simulink model "MSM_strain_wave_actuator"  (R2024b)
settings: Solver=ode23t  StartTime=0.0  StopTime=SIMULATION_TIME  FixedStep=MAX_TIME_STEP  MaxStep=MAX_TIME_STEP  RelTol=1e-3  AbsTol=1e-3  EnableMultiTasking=on
PreLoadFcn:
  | linear_mechanism = Simulink.Variant('motion_type == "linear"');
  | rotary_mechanism = Simulink.Variant('motion_type == "rotary"');
values from neighbouring files (symbols this model uses):
  action = round(out.position_data.Data(:,5))    [msm_tooth_training_run.m]
  contact_ratio = tooth_plates_cnt / (2 * (t_a / t_b + 1))    (= 2)    [MSM_mechanism_simulation_properties.m]
  contraction_initial = -msm_length * e_initial    (= -0.001)    [MSM_mechanism_simulation_properties.m]
  controller_type_vec = zeros(tooth_plates_cnt, 1)    [MSM_mechanism_simulation_properties.m]
  controller_velocity_setpoint = velocity_iter    [controller_mass_comparison_runs.m]
  disk_diameter = disk_teeth_count * tooth_pitch / pi    [MSM_mechanism_simulation_properties.m]    (also in msm_sim_runs_for_pid.m = evalin('base','disk_diameter'); save_sim_result.m = evalin('base','disk_diameter'))
  disk_height = 2.5e-4    (= 0.00025)    [MSM_mechanism_simulation_properties.m]    (also in get_tooth_properties.m)
  feedback_threshold = 1.025    [MSM_mechanism_simulation_properties.m]    (also in get_tooth_properties.m; msm_sim_runs_for_pid.m = evalin('base','feedback_threshold'))
  force_control_coeff = 1.0    (= 1)    [MSM_mechanism_simulation_properties.m]
  HALT_VELOCITY = 0.2    [MSM_mechanism_simulation_properties.m]    (also in get_tooth_properties.m)
  in_pair_angle_tooth_plates_pitch = 2*pi * (-2*tooth_pitch + in_pair_tooth_plates_pitch) / (pi*disk_diameter)    (= 0.412285714286)    [MSM_mechanism_simulation_properties.m]    (also in get_tooth_properties.m = 2*pi * (-2*tooth_pitch + in_pair_tooth_plates_pitch) / (pi*t)
  MAX_OVERLOAD_VELOCITY = 100    [MSM_mechanism_simulation_properties.m]    (also in get_tooth_properties.m)
  MAX_POSITION = rack_initial_position + max_teeth_passed * tooth_plates_cnt * angle_single_tooth_step    [MSM_mechanism_simulation_properties.m]    (also in get_tooth_properties.m)
  MAX_TIME_STEP = 5e-6    (= 5e-06)    [MSM_mechanism_simulation_properties.m]
  min_tooth_motion_range = -msm_length * allowed_elongation    (= -0.001)    [MSM_mechanism_simulation_properties.m]
  motion_type_number = NaN    [MSM_mechanism_simulation_properties.m]
  next_vec_fraction = -0.05    [MSM_mechanism_simulation_properties.m]    (also in msm_sim_runs_for_pid.m = evalin('base','next_vec_fraction'))
  obs_matrix = zeros(tooth_plates_cnt, obs_matrix_size)    [MSM_mechanism_simulation_properties.m]
  one_side_absolute_offset = one_side_elongation_capacity * msm_length    (= 0.0001)    [MSM_mechanism_simulation_properties.m]
  rack_coulumb_friction = 0.05    [MSM_mechanism_simulation_properties.m]
  rack_initial_position = rack_initial_position + 4*angle_single_tooth_step    (= 0.0554357142857)    [MSM_mechanism_simulation_properties.m]    (also in get_tooth_properties.m = rack_initial_position + 4*angle_single_tooth_step)
  rack_mass = 4e-3    (= 0.004)    [MSM_mechanism_simulation_properties.m]
  rotational_rack_coulumb_friction = rack_coulumb_friction * disk_diameter    (= 0.00175)    [MSM_mechanism_simulation_properties.m]
  SIMULATION_TIME = 0.06    [MSM_mechanism_simulation_properties.m]    (also in msm_actuation_time_sensetivity.m = 0.04; msm_sim_runs_for_pid.m = evalin('base','SIMULATION_TIME'); msm_simulation_run.m = 0.08; msm_tooth_training_run.m = 0.04)
  swing_block_tooth_plates_pitch = 2 * tooth_pitch * 22 + tooth_pitch / tooth_plates_cnt    (= 0.0172575)    [MSM_mechanism_simulation_properties.m]    (also in get_tooth_properties.m = 2 * tooth_pitch * 22 + tooth_pitch / tooth_plates_cnt)
  tooth_disk_mass = 5e-3    (= 0.005)    [MSM_mechanism_simulation_properties.m]
  tooth_pitch = tooth_pitch * tooth_size_modifier    (= 0.00039)    [MSM_mechanism_simulation_properties.m]    (also in get_tooth_properties.m = 0.00024661; msm_sim_runs_for_pid.m = evalin('base','tooth_pitch'); save_sim_result.m = evalin('base','tooth_pitch'))
  tooth_plates_cnt = 4    [MSM_mechanism_simulation_properties.m]    (also in MSM_simulation_data_processing.m = sim_data.tooth_plates_cnt; msm_actuation_time_sensetivity.m = plates_cnt_iter; msm_sim_runs_for_pid.m = evalin('base','tooth_plates_cnt'); msm_simulation_run.m = plates_cnt_iter)
  tooth_plates_pitch = tooth_pitch * 12 + tooth_pitch / tooth_plates_cnt    (= 0.0047775)    [MSM_mechanism_simulation_properties.m]    (also in get_tooth_properties.m = tooth_pitch * 12 + tooth_pitch / tooth_plates_cnt)
  useful_load = -2    [MSM_mechanism_simulation_properties.m]    (also in controller_mass_comparison_runs.m)
  useful_mass = 0.0001    [MSM_mechanism_simulation_properties.m]    (also in controller_mass_comparison_runs.m = 0.025)
  VALIDATION_START_TIME = 0.25*SIMULATION_TIME    (= 0.015)    [MSM_mechanism_simulation_properties.m]
  Z = griddata(x,y,z,X,Y)    [MSM_simulation_data_processing.m]
undefined symbols (not defined in the file or in its folder): controller_amplitude_setpoint, controller_desired_profile_type, controller_frequency_setpoint, controller_loop_type, enable_neighbours_obs, enable_vel_setpoint, external_control_value, has_external_controller, initial_spike_force, random_delay_probablity, random_switch_probability, sim_state_code, simulation_pause_time, X, Y
libraries: sm_lib x141, MSM_element x72, Flat_tooth_plate x36, Rotary_tooth_plate x36, Swing_mechanism x18, nesl_utility x16, simulink x10, fl_lib x9, rllib x7, spsMeanLib x2, slctrl_autotuning x2, slpidlib x1
(part 2 of 7)

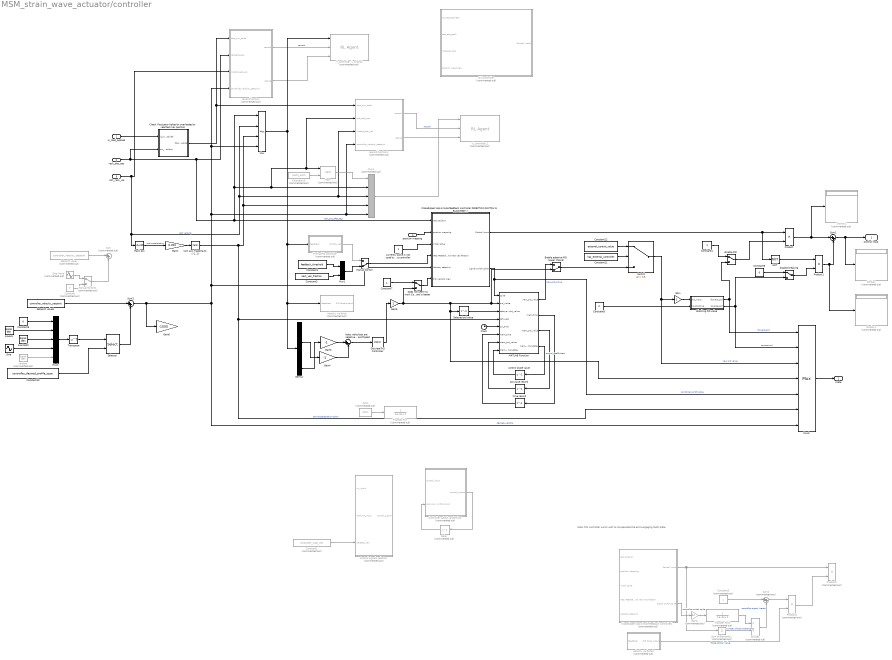
== system MSM_strain_wave_actuator/controller ==
  note: Note: this controller works well to compensate the extra engaging tooth plate
  is_load_applied : Inport
  rack_abs_pos : Inport  Port=2
  inst_rack_vel : Inport  Port=3
  position mapping : Inport  Port=4
  Blocking PID value : MATLAB Function  TreatAsAtomicUnit=on
  Check if actuator halted or overloaded or reached max position : Subsystem
  Clock : Clock
  Closed/open loop simple feedback controller DIRECTION SWITCH IS BLOCKED!!!! : Subsystem
  Closed/open loop simple feedback controller1 : Subsystem  Commented=on
  Constant : Constant  Commented=on  Value=0
  Constant1 : Constant  Value=feedback_threshold
  Constant10 : Constant  Value=controller_desired_profile_type
  Constant11 : Constant  Value=has_external_controller
  Constant12 : Constant  Value=external_control_value
  Constant13 : Constant  Commented=on  Value=tooth_pitch
  Constant2 : Constant  Commented=on  Value=controller_type_vec
  Constant3 : Constant  Value=next_vec_fraction
  Constant4 : Constant
  Constant5 : Constant  Commented=on
  Constant6 : Constant  Value=0
  Constant7 : Constant
  Constant8 : Constant  Value=0
  Constant9 : Constant  Value=0
  Control signals selector : MATLAB Function  Commented=on  TreatAsAtomicUnit=on
  Controller output randomizer : MATLAB Function  Commented=on  TreatAsAtomicUnit=on
  Delay : Delay  Commented=on  DelayLength=1  InitialCondition=zeros(tooth_plates_cnt, 1)
  Delayed pid value : Delay
  Demux : Demux
  "Discrete PID Controller " : slpidlib/PID Controller  Controller=PID  Form=Parallel  TimeDomain=Discrete-time  UseExternalTs=off  SampleTime=1/2000  IntegratorMethod=Forward Euler  FilterMethod=Forward Euler  ControllerParametersSource=internal  P=6  I=2e+4  UseKiTs=off  D=8e-5  UseExternalDerivativeSource=off  N=100  UseFilter=off  TunerSelectOption=Transfer Function Based (PID Tuner App)  InitialConditionSource=internal  InitialConditionForIntegrator=0  InitialConditionForFilter=0  DifferentiatorICPrevScaledInput=0  ExternalReset=none  TrackingMode=off  Kt=1  LimitOutput=off  SatLimitsSource=internal  UpperSaturationLimit=inf  LowerSaturationLimit=-inf  LinearizeAsGain=off  AntiWindupMode=none  Kb=1  LimitIntegrator=off  UpperIntegratorSaturationLimit=inf  LowerIntegratorSaturationLimit=-inf  POutMin=[]  POutMax=[]  IOutMin=[]  IOutMax=[]  DOutMin=[]  DOutMax=[]  NOutMin=[]  NOutMax=[]  SumOutMin=[]  SumOutMax=[]  SaturationOutMin=[]  SaturationOutMax=[]  PParamMin=[]  PParamMax=[]  IParamMin=[]  IParamMax=[]  DParamMin=[]  DParamMax=[]  NParamMin=[]  NParamMax=[]  KbParamMin=[]  KbParamMax=[]  KtParamMin=[]  KtParamMax=[]  KbOutMin=[]  KbOutMax=[]  KtOutMin=[]  KtOutMax=[]  IntegratorOutMin=[]  IntegratorOutMax=[]  FilterOutMin=[]  FilterOutMax=[]  SumI1OutMin=[]  SumI1OutMax=[]  SumI2OutMin=[]  SumI2OutMax=[]  SumI3OutMin=[]  SumI3OutMax=[]  SumI4OutMin=[]  SumI4OutMax=[]  SumDOutMin=[]  SumDOutMax=[]  DifferentiatorOutMin=[]  DifferentiatorOutMax=[]  FilterDiffOutCoefMin=[]  FilterDiffOutCoefMax=[]  ReciprocalOutMin=[]  ReciprocalOutMax=[]  SumDenOutMin=[]  SumDenOutMax=[]  SumNumOutMin=[]  SumNumOutMax=[]  DivideOutMin=[]  DivideOutMax=[]  UdiffTsProdOutMin=[]  UdiffTsProdOutMax=[]  NTsProdOutMin=[]  NTsProdOutMax=[]  UintegralTsProdOutMin=[]  UintegralTsProdOutMax=[]  UngainTsProdOutMin=[]  UngainTsProdOutMax=[]  ClampingZeroOutDataTypeStr=Inherit: Inherit via back propagation  ClampingZeroOutMin=[]  ClampingZeroOutMax=[]  FilterDenConstantOutDataTypeStr=Inherit: Inherit via back propagation  FilterDenConstantOutMin=[]  FilterDenConstantOutMax=[]  PCopyOutDataTypeStr=Inherit: Inherit via back propagation  PCopyOutMin=[]  PCopyOutMax=[]  NCopyOutDataTypeStr=Inherit: Inherit via back propagation  NCopyOutMin=[]  NCopyOutMax=[]  IntegratorContinuousStateAttributes=''  IntegratorStateMustResolveToSignalObject=off  IntegratorRTWStateStorageClass=Auto  FilterContinuousStateAttributes=''  FilterStateMustResolveToSignalObject=off  FilterRTWStateStorageClass=Auto  ParallelPVariant=InternalParameters  IdealPVariant=Disabled  IVariant=InternalParameters  DVariant=InternalParameters  IntegratorVariant=Discrete  SatVariant=Disabled  AWVariant=Passthrough  PCopyVariant=Disabled  TRVariant=Disabled  FdbkBlocksVariant=Forward  IdealPFdbkVariant=Disabled  SatFdbkVariant=Disabled  DerivativeFilterVariant=Differentiator  NVariant=Passthrough  NCopyVariant=Disabled_SignalSpec  FilterICVariant=InternalICsDifferentiator  IntegratorICVariant=InternalICs  ExternalResetVariant=Disabled  TRSumVariant=Passthrough  SumFdbkVariant=Disabled  SumVariant=Sum_PID  TsampFilterVariant=InternalTs  TsampNgainVariant=Passthrough  TsampIntegralVariant=Disabled_SignalSpec  ExternalSaturationOutDataTypeStr=Inherit: Same as second input  DerivativeSourceVariant=ErrorSignal  PreIntVariant=InternalPreInt
      settings: LibrarySourceBlock=simulink/Discrete/Discrete PID Controller
  Display : Display  Commented=on
  Display1 : Display  Commented=on
  Display2 : Display  Commented=on
  Divide1 : Product  Commented=on  Inputs=*/
  Does not seem to work Constant is better : ManualSwitch
  Enable adaptive PID (upper choice) : ManualSwitch  CurrentSetting=0
  Gain : Gain
  Gain1 : Gain  Gain=0.001
  Gain2 : Gain  Commented=on  Gain=32
  Gain3 : Gain  Gain=-1
  Gain4 : Gain  Gain=-1
  Gain5 : Gain
  Gain6 : Gain  Gain=-1000
  MATLAB Function : MATLAB Function  TreatAsAtomicUnit=on
  Manual Switch : ManualSwitch  CurrentSetting=0
  Manual Switch1 : ManualSwitch  Commented=on
  Mux : Mux
  Mux1 : Mux  Inputs=2
  Mux2 : Mux  Inputs=5
  Mux3 : Mux  Inputs=7
  Mux4 : Mux  Commented=on  Inputs=5
  NOT : Logic  Operator=NOT  IconShape=distinctive  AllPortsSameDT=off  OutDataTypeStr=boolean
  Note: velocities are negative but output is positive that is why the input signs are flipped : Sum  Inputs=|+-
  Old controller : Subsystem  Commented=on
  PWM : simulink/Discontinuities/PWM  Commented=on  DisableCoverage=on  Period=1 / 2e+4  InitialDelay=0  DisallowZeroDutyCycle=off  RunAtFixedTimeIntervals=off  SampleTime=0.1
  Product : Product
  Product1 : Product
  Product2 : Product  Commented=on
  Product3 : Product  Commented=on
  Rack acc : Derivative
  Rem : Math  Commented=on  Operator=rem
  Selector : Selector  InputPortWidth=5  IndexOptions=Index vector (port)  Indices=[1 3]  OutputSizes=1
  Setpoint value : Constant  Commented=on  Value=controller_velocity_setpoint
  Setpoint value1 : Constant  Value=controller_velocity_setpoint
  Sine : Sin  Amplitude=controller_amplitude_setpoint  Frequency=controller_frequency_setpoint  Phase=pi*0  SampleTime=0
  Sine Wave : Sin  Commented=on  Amplitude=-0.01  Frequency=350  Phase=pi*0  SampleTime=0
  Sum : Sum  Commented=on  Inputs=|++
  Sum of Elements1 : Sum  Commented=on  Inputs=+
  Sum1 : Sum  Inputs=|++
  Sum2 : Sum  Commented=on  Inputs=|++
  Sum3 : Sum  Inputs=|++
  Switch : Switch  Criteria=u2 > Threshold  Threshold=0.5  SaturateOnIntegerOverflow=off  InputSameDT=off
  Timing PID controller : Subsystem  Commented=on
  Transfer Fcn : TransferFcn  Commented=on  Denominator=[1e-4 1]
  Transfer Fcn2 : TransferFcn  Commented=on  Denominator=[1e-4 1]
  Transpose : Math  Operator=transpose
  control state value : Delay  DelayLength=1
  currently spike is not used by the controller : Constant
  disable PID : ManualSwitch
  disable breaking : ManualSwitch
  pid value record : Delay  DelayLength=1
  "rack acc mapping to [-1, 1]" : Trigonometry  Operator=tanh
  random : SignalGenerator  Commented=on  WaveForm=random  Amplitude=controller_amplitude_setpoint  Frequency=controller_frequency_setpoint  Units=rad/sec
  reward function : MATLAB Function  Commented=on  TreatAsAtomicUnit=on
  reward function1 : MATLAB Function  Commented=on  TreatAsAtomicUnit=on
  rl_controller_1 : rllib/RL Agent  Commented=on  Agent=agent  ExternalActionAsInput=off  ProvideLastAction=off  ProvideCumRwd=off  TreatAsDirectFeedthrough=on  UseStrictObservationDataTypes=off
  rl_controller_1_original : rllib/RL Agent  Commented=on  Agent=agent  ExternalActionAsInput=off  ProvideLastAction=off  ProvideCumRwd=off  TreatAsDirectFeedthrough=on  UseStrictObservationDataTypes=off
  sawtooth : SignalGenerator  WaveForm=sawtooth  Amplitude=controller_amplitude_setpoint  Frequency=controller_frequency_setpoint  Units=rad/sec
  square : SignalGenerator  WaveForm=square  Amplitude=controller_amplitude_setpoint  Frequency=controller_frequency_setpoint  Units=rad/sec
  time record : Delay  DelayLength=1
  velocity via force : Subsystem  Commented=on
  velocity via force1 : Subsystem  Commented=on
  Control input : Outport
  state : Outport  Port=2
  wires:
  Check if actuator halted or overloaded or reached max position/1(stop_sim_code) -> reward function/1(stop_sim_code), reward function1/1(stop_sim_code)
  reward function/1(reward) -> rl_controller_1_original/2  "reward"
  position mapping/1 -> Closed/open loop simple feedback controller DIRECTION SWITCH IS BLOCKED!!!!/2(position mapping)
  reward function/2(isdone) -> rl_controller_1_original/3
  inst_rack_vel/1 -> reward function/3(instant_rack_vel), reward function1/3(instant_rack_vel), Mux4/3, Mux/2, Rack acc/1  "rack velocity"
  rack_abs_pos/1 -> Check if actuator halted or overloaded or reached max position/2(cur_rack_position), reward function1/2(rack_abs_pos), Rem/1, Mux4/2, Mux/1, Closed/open loop simple feedback controller DIRECTION SWITCH IS BLOCKED!!!!/1(rack position), reward function/2(rack_abs_pos)  "rack_pos_after_tag"
  "rack acc mapping to [-1, 1]"/1 -> Mux3/6, MATLAB Function/4(tahn_acc), Mux4/4, Mux/3  "tanh(accelecration*1e-3)"
  is_load_applied/1 -> Check if actuator halted or overloaded or reached max position/1(is_load_applied)
  currently spike is not used by the controller/1 -> Closed/open loop simple feedback controller DIRECTION SWITCH IS BLOCKED!!!!/3(initial spike)
  Constant2/1 -> Control signals selector/3(selector_vec)
  Controller output randomizer/1(control_output) -> Delay/1
  Delay/1 -> Controller output randomizer/2(previous_control_input)
  Rack acc/1 -> Gain1/1  "rack acceleration"
  Gain1/1 -> "rack acc mapping to [-1, 1]"/1
  Constant3/1 -> Mux1/2
  Constant1/1 -> Mux1/1
  Mux1/1 -> Manual Switch/2
  Timing PID controller/1(control_vec) -> Manual Switch/1
  Manual Switch/1 -> Closed/open loop simple feedback controller DIRECTION SWITCH IS BLOCKED!!!!/4(VEC: Feedback threshold and next vec fraction)
  PWM/1 -> Transfer Fcn/1
  Setpoint value/1 -> Sum/1
  Sine Wave/1 -> Manual Switch1/1
  Constant/1 -> Manual Switch1/2
  Manual Switch1/1 -> Sum/2
  Closed/open loop simple feedback controller DIRECTION SWITCH IS BLOCKED!!!!/2(signal switch spike) -> Mux3/5, MATLAB Function/1(spike)  "controller switch spike"
  Divide1/1 -> Sum2/2  "controller signal inertia"
  Product3/1 -> Product2/2
  Sum of Elements1/1 -> Divide1/2  "number of active elements"
  Sum2/1 -> Product3/1
  Transfer Fcn2/1 -> Divide1/1
  Constant5/1 -> Sum2/1
  Gain2/1 -> Transfer Fcn2/1
  Closed/open loop simple feedback controller1/2(signal switch spike) -> Gain2/1  "controller switch spike"
  velocity via force1/1(PID force output) -> Product3/2  "Force control value"
  Closed/open loop simple feedback controller1/1(Control Input) -> Sum of Elements1/1, Product2/1
  pid value record/1 -> MATLAB Function/7("mem_pid_value ")
  MATLAB Function/3(mem_pid_value) -> pid value record/1
  time record/1 -> MATLAB Function/6("mem_time ")
  MATLAB Function/2(mem_time) -> time record/1
  Clock/1 -> MATLAB Function/5(cur_time)
  Delayed pid value/1 -> MATLAB Function/3(delayed_pid_value)
  MATLAB Function/4(mem_control_state) -> control state value/1  "control_coefficitent"
  control state value/1 -> MATLAB Function/8("mem_control_state ")
  disable PID/1 -> Product/2
  Constant4/1 -> disable PID/1
  Closed/open loop simple feedback controller DIRECTION SWITCH IS BLOCKED!!!!/1(Control Input) -> Product/1, NOT/1
  NOT/1 -> Product1/1
  Product/1 -> Display2/1, Sum1/1
  Product1/1 -> Display1/1, Sum1/2
  Sum1/1 -> Display/1, Control input/1
  Constant6/1 -> disable breaking/1
  disable breaking/1 -> Product1/2
  Constant7/1 -> Does not seem to work Constant is better/1
  Does not seem to work Constant is better/1 -> Closed/open loop simple feedback controller DIRECTION SWITCH IS BLOCKED!!!!/6(PID velocity sign)
  Blocking PID value/1(forward_pid) -> Mux3/1, disable PID/2  "forward_pid"
  Blocking PID value/2(reverse_pid) -> Mux3/2, disable breaking/2  "reverse pid"
  Constant8/1 -> Blocking PID value/2(no_blocking)
  Setpoint value1/1 -> Sum3/1
  Selector/1 -> Sum3/2
  Sum3/1 -> Gain6/1, Mux3/7, Mux/4, reward function/4(controller_velocity_setpoint), reward function1/4(controller_velocity_setpoint), Mux4/5, Closed/open loop simple feedback controller DIRECTION SWITCH IS BLOCKED!!!!/5(Velocity setpoint)  "desired_velocity"
  Mux2/1 -> Transpose/1
  square/1 -> Mux2/2
  sawtooth/1 -> Mux2/3
  Constant10/1 -> Selector/2
  Constant9/1 -> Mux2/1
  Transpose/1 -> Selector/1
  Sine/1 -> Mux2/4
  random/1 -> Mux2/5
  Mux3/1 -> state/1
  Switch/1 -> Mux3/3, Gain/1  "new pid value"
  MATLAB Function/1(new_pid_value) -> Enable adaptive PID (upper choice)/1  "new_pid_value"
  Constant11/1 -> Switch/2
  Constant12/1 -> Switch/1
  Mux4/1 -> rl_controller_1/1
  Constant13/1 -> Rem/2
  Rem/1 -> Mux4/1
  reward function1/2(isdone) -> rl_controller_1/3
  reward function1/1(reward) -> rl_controller_1/2  "reward"
  Gain/1 -> Blocking PID value/1(pid_input)
  Mux/1 -> Timing PID controller/1(feedback), Demux/1, velocity via force/1(feedback), rl_controller_1_original/1
  Gain3/1 -> Note: velocities are negative but output is positive that is why the input signs are flipped/1
  Demux/4 -> Gain3/1
  Demux/2 -> Gain4/1
  Gain4/1 -> Note: velocities are negative but output is positive that is why the input signs are flipped/2
  Note: velocities are negative but output is positive that is why the input signs are flipped/1 -> "Discrete PID Controller "/1
  Gain5/1 -> Mux3/4, Delayed pid value/1, Enable adaptive PID (upper choice)/2, MATLAB Function/2(pid_value), Does not seem to work Constant is better/2
  "Discrete PID Controller "/1 -> Gain5/1
  Enable adaptive PID (upper choice)/1 -> Switch/3

== system MSM_strain_wave_actuator/MSM elements variant subsystem/Variable plate count Linear push push plates ==
  Control input : Inport
  Linear_swing_eight_tooth_plates : Subsystem  VariantControl=eight_tooth_plates
  Linear_swing_four_tooth_plates : Subsystem  VariantControl=four_tooth_plates
  Linear_swing_six_tooth_plates : Subsystem  VariantControl=six_tooth_plates
  Frame : PMIOPort  Side=Left
  Spatial force output : PMIOPort  Port=2  Side=Right
  Position Feedback : Outport
  Data output : Outport  Port=2

== system MSM_strain_wave_actuator/MSM elements variant subsystem/Variable plate count Rotary push push plates ==
  Control input : Inport
  Rotary push push 4 plates : Subsystem  VariantControl=four_tooth_plates
  Rotary push push 6 plates : Subsystem  VariantControl=six_tooth_plates
  Rotary push push 8 plates : Subsystem  VariantControl=eight_tooth_plates
  Frame : PMIOPort  Side=Left
  Spatial force output : PMIOPort  Port=2  Side=Right
  Position Feedback : Outport
  Data output : Outport  Port=2

== system MSM_strain_wave_actuator/MSM elements variant subsystem/Variable plate count Rotary push spring plates ==
  Control input : Inport
  Rotary push spring 4 plates : Subsystem  VariantControl=four_tooth_plates
  Rotary push spring 6 plates : Subsystem  VariantControl=six_tooth_plates
  Rotary push spring 8 plates : Subsystem  VariantControl=eight_tooth_plates
  Frame : PMIOPort  Side=Left
  Spatial force output : PMIOPort  Port=2  Side=Right
  Position Feedback : Outport
  Data output : Outport  Port=2

== system MSM_strain_wave_actuator/MSM elements variant subsystem/Variable plate count Spring returned plates ==
  Control input : Inport
  eight_tooth_plates : Subsystem  VariantControl=eight_tooth_plates
  four_tooth_plates : Subsystem  VariantControl=four_tooth_plates
  six_tooth_plates : Subsystem  VariantControl=six_tooth_plates
  Frame : PMIOPort  Side=Left
  Spatial force output : PMIOPort  Port=2  Side=Right
  Position Feedback : Outport
  Data output : Outport  Port=2

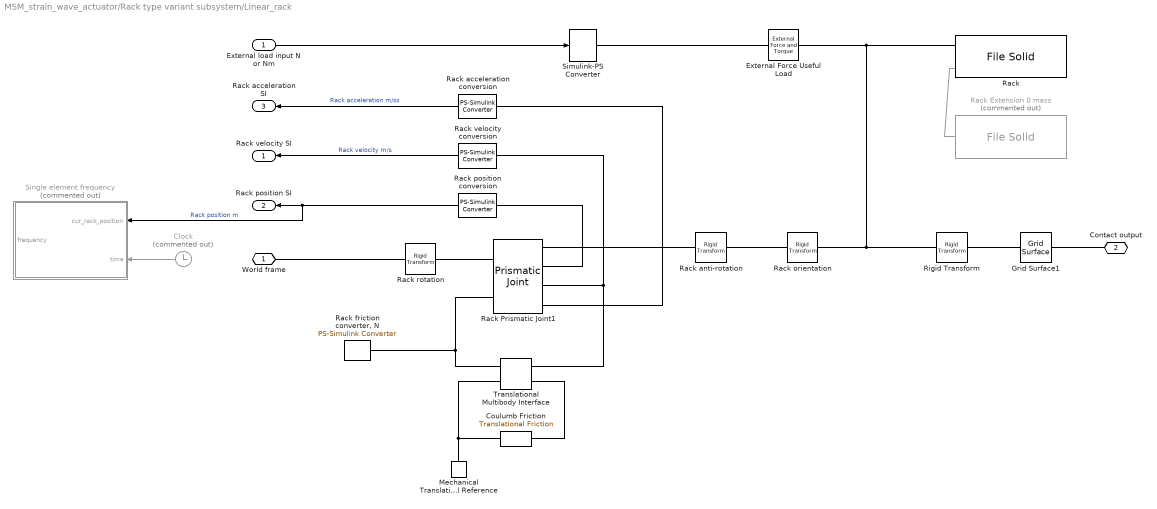
== system MSM_strain_wave_actuator/Rack type variant subsystem/Linear_rack ==
  External load input N or Nm : Inport
  Clock : Clock  Commented=on
  Coulumb Friction : fl_lib/Mechanical/Translational Elements/Translational Friction  brkwy_frc=rack_coulumb_friction * (1 + 1e-5) N  brkwy_vel=1e-2 m/s  Col_frc=rack_coulumb_friction N  visc_coef=bronze_steel_kinetic_friction N*s/m  v_specify=off  v_priority=None  v=0 m/s  v_nominal_specify=off  v_nominal_value=1  v_nominal_unit=m/s  f_specify=off  f_priority=None  f=0 N  f_nominal_specify=off  f_nominal_value=1  f_nominal_unit=N
      settings: InternalSimscapePortConfiguration="{\"Bottom\":[],\"Left\":[{\"id\":\"R\",\"label\":\"R\",\"type\":\"foundation.mechanical.translational.translational\"}],\"Right\":[{\"id\":\"C\",\"label\":\"C\",\"type\":\"foundation.mechanical.translational.translational\"}],\"Top\":[]}"
  External Force Useful Load : sm_lib/Forces and Torques/External Force and Torque  EnableForceX=on  EnableForceY=off  EnableForceZ=off  EnableForce=off  ForceResolutionFrame=World  EnableTorqueX=off  EnableTorqueY=off  EnableTorqueZ=off  EnableTorque=off  TorqueResolutionFrame=AttachedFrame
  Grid Surface1 : sm_lib/Curves and Surfaces/Grid Surface  XGridVector=x_grid_vec  XGridVectorUnits=m  YGridVector=rack_y_grid  YGridVectorUnits=m  ZHeights=rack_z_grid  ZHeightsUnits=m  GraphicType=FromGeometry  GraphicVisPropType=SimpleVisualProperties  GraphicDiffuseColor=[1 0.4118 0.1608]  GraphicOpacity=1.0  GraphicSpecularColor=[0.5 0.5 0.5 1.0]  GraphicAmbientColor=[0.15 0.15 0.15 1.0]  GraphicEmissiveColor=[0.0 0.0 0.0 1.0]  GraphicShininess=75
  Mechanical Translational Reference : fl_lib/Mechanical/Translational Elements/Mechanical Translational Reference
  Rack : sm_lib/Body Elements/File Solid  ExtGeomFileName=Rack.STEP  UnitType=FromFile  ExtGeomFileUnits=m  StepReaderType=HEX  ExportConvexHullGeometry=off  InertiaType=CalculateFromGeometry  BasedOnType=Mass  Density=1000  DensityUnits=kg/m^3  Mass=rack_mass+useful_mass  MassUnits=kg  CenterOfMass=[0 0 0]  CenterOfMassUnits=m  MomentsOfInertia=[1 1 1]  MomentsOfInertiaUnits=kg*m^2  ProductsOfInertia=[0 0 0]  ProductsOfInertiaUnits=kg*m^2  GraphicType=FromGeometry  MarkerShape=Sphere  MarkerSize=10  GraphicVisPropType=SimpleVisualProperties  GraphicDiffuseColor=[1.0 0.8 0.4]  GraphicOpacity=solid_block_opacity  GraphicSpecularColor=[0.5 0.5 0.5 1.0]  GraphicAmbientColor=[0.15 0.15 0.15 1.0]  GraphicEmissiveColor=[0.0 0.0 0.0 1.0]  GraphicShininess=75  DoExposeReferenceFrame=off  SerializedFrames=<Frames><Frame><Id>Frame1</Id><Value><Name>Edge center</Name><Origin><Source>GeometricFeature</Source><FeatureName>segment 567</FeatureName></Origin><PrimaryAxis><DefinedDirection>+Z</DefinedDirection><Source>ReferenceFrame</Source><SourceDirection>+Z</SourceDirection><FeatureName></FeatureName></PrimaryAxis><SecondaryAxis><DefinedDirection>+X</DefinedDirection><Source>ReferenceFrame</Source><SourceDirection>+X</SourceDirection><FeatureName></FeatureName></SecondaryAxis></Value></Frame><Frame><Id>Frame2</Id><Value><Name>Staqck_Out</Name><Origin><Source>GeometricFeature</Source><FeatureName>segment 578</FeatureName></Origin><PrimaryAxis><DefinedDirection>+Z</DefinedDirection><Source>ReferenceFrame</Source><SourceDirection>+Z</SourceDirection><FeatureName></FeatureName></PrimaryAxis><SecondaryAxis><DefinedDirection>+X</DefinedDirection><Source>ReferenceFrame</Source><SourceDirection>+X</SourceDirection><FeatureName></FeatureName></SecondaryAxis></Value></Frame><Frame><Id>Frame3</Id><Value><Name>Stack_In</Name><Origin><Source>GeometricFeature</Source><FeatureName>segment 2239</FeatureName></Origin><PrimaryAxis><DefinedDirection>+Z</DefinedDirection><Source>ReferenceFrame</Source><SourceDirection>+Z</SourceDirection><FeatureName></FeatureName></PrimaryAxis><SecondaryAxis><DefinedDirection>+X</DefinedDirection><Source>ReferenceFrame</Source><SourceDirection>+X</SourceDirection><FeatureName></FeatureName></SecondaryAxis></Value></Frame></Frames>
  Rack Extension 0 mass : sm_lib/Body Elements/File Solid  Commented=on  ExtGeomFileName=Rack.STEP  UnitType=FromFile  ExtGeomFileUnits=m  StepReaderType=HEX  ExportConvexHullGeometry=off  InertiaType=CalculateFromGeometry  BasedOnType=Mass  Density=1000  DensityUnits=kg/m^3  Mass=1e-10  MassUnits=kg  CenterOfMass=[0 0 0]  CenterOfMassUnits=m  MomentsOfInertia=[1 1 1]  MomentsOfInertiaUnits=kg*m^2  ProductsOfInertia=[0 0 0]  ProductsOfInertiaUnits=kg*m^2  GraphicType=FromGeometry  MarkerShape=Sphere  MarkerSize=10  GraphicVisPropType=SimpleVisualProperties  GraphicDiffuseColor=[1.0 0.8 0.4]  GraphicOpacity=solid_block_opacity  GraphicSpecularColor=[0.5 0.5 0.5 1.0]  GraphicAmbientColor=[0.15 0.15 0.15 1.0]  GraphicEmissiveColor=[0.0 0.0 0.0 1.0]  GraphicShininess=75  DoExposeReferenceFrame=off  SerializedFrames=<Frames><Frame><Id>Frame1</Id><Value><Name>Edge center</Name><Origin><Source>GeometricFeature</Source><FeatureName>segment 567</FeatureName></Origin><PrimaryAxis><DefinedDirection>+Z</DefinedDirection><Source>ReferenceFrame</Source><SourceDirection>+Z</SourceDirection><FeatureName></FeatureName></PrimaryAxis><SecondaryAxis><DefinedDirection>+X</DefinedDirection><Source>ReferenceFrame</Source><SourceDirection>+X</SourceDirection><FeatureName></FeatureName></SecondaryAxis></Value></Frame><Frame><Id>Frame2</Id><Value><Name>Staqck_Out</Name><Origin><Source>GeometricFeature</Source><FeatureName>segment 578</FeatureName></Origin><PrimaryAxis><DefinedDirection>+Z</DefinedDirection><Source>ReferenceFrame</Source><SourceDirection>+Z</SourceDirection><FeatureName></FeatureName></PrimaryAxis><SecondaryAxis><DefinedDirection>+X</DefinedDirection><Source>ReferenceFrame</Source><SourceDirection>+X</SourceDirection><FeatureName></FeatureName></SecondaryAxis></Value></Frame><Frame><Id>Frame3</Id><Value><Name>Stack_In</Name><Origin><Source>GeometricFeature</Source><FeatureName>segment 2239</FeatureName></Origin><PrimaryAxis><DefinedDirection>+Z</DefinedDirection><Source>ReferenceFrame</Source><SourceDirection>+Z</SourceDirection><FeatureName></FeatureName></PrimaryAxis><SecondaryAxis><DefinedDirection>+X</DefinedDirection><Source>ReferenceFrame</Source><SourceDirection>+X</SourceDirection><FeatureName></FeatureName></SecondaryAxis></Value></Frame></Frames>
  Rack Prismatic Joint1 : sm_lib/Joints/Prismatic Joint  JointMode=Normal  CompositeWrenchDir=FollowerOnBase  CompositeWrenchFrame=BaseFrame  SenseConstraintForce=off  SenseConstraintTorque=off  SenseTotalForce=off  SenseTotalTorque=off  PositionTargetSpecify=on  PositionTargetPriority=High  PositionTargetValue=rack_initial_position  PositionTargetValueUnits=m  VelocityTargetSpecify=on  VelocityTargetPriority=High  VelocityTargetValue=rack_initial_velocity  VelocityTargetValueUnits=m/s  EquilibriumPosition=0  EquilibriumPositionUnits=m  SpringStiffness=0  SpringStiffnessUnits=N/m  DampingCoefficient=0  DampingCoefficientUnits=N/(m/s)  LowerLimitSpecify=off  LowerLimitBound=-1  LowerLimitBoundUnits=m  LowerLimitStiffness=1e6  LowerLimitStiffnessUnits=N/m  LowerLimitDamping=1e3  LowerLimitDampingUnits=N/(m/s)  LowerLimitTransitionRegionWidth=1e-4  LowerLimitTransitionRegionWidthUnits=m  UpperLimitSpecify=off  UpperLimitBound=1  UpperLimitBoundUnits=m  UpperLimitStiffness=1e6  UpperLimitStiffnessUnits=N/m  UpperLimitDamping=1e3  UpperLimitDampingUnits=N/(m/s)  UpperLimitTransitionRegionWidth=1e-4  UpperLimitTransitionRegionWidthUnits=m  TorqueActuationMode=InputTorque  MotionActuationMode=ComputedMotion  SensePosition=on  SenseVelocity=on  SenseAcceleration=on  SenseTorqueForce=off  SenseLowerLimitTorqueForce=off  SenseUpperLimitTorqueForce=off
  Rack acceleration conversion : nesl_utility/PS-Simulink Converter  PhysicalDomain=network_engine_domain  SubClassName=ps_output  LeftPortType=input  RightPortType=output  PseudoPeriodic=off  Frequencies=[]  VectorFormat=inherit  Unit=inherit  AffineConversion=off
  Rack anti-rotation : sm_lib/Frames and Transforms/Rigid Transform  RotationMethod=StandardAxis  FollAlignAxisA=+X  BaseAlignAxisA=+Y  FollAlignAxisB=+Y  BaseAlignAxisB=+Z  RotationStandardAxis=-Y  RotationAngle=-90.0  RotationAngleUnits=deg  RotationArbitraryAxis=[0 0 1]  RotationSequenceAxes=FollowerAxes  RotationSequence=XYX  RotationSequenceAngles=[0 0 0]  RotationSequenceAnglesUnits=deg  RotationMatrix=[1 0 0; 0 1 0; 0 0 1]  Quaternion=[1 0 0 0]  TranslationMethod=None  TranslationCartesianOffset=[0 0 0]  TranslationCartesianOffsetUnits=m  TranslationStandardAxis=+Z  TranslationStandardOffset=0  TranslationStandardOffsetUnits=m  TranslationROffset=0  TranslationROffsetUnits=m  TranslationThetaOffset=0  TranslationThetaOffsetUnits=deg  TranslationZOffset=0  TranslationZOffsetUnits=m
  "Rack friction converter, N" : nesl_utility/PS-Simulink Converter  PhysicalDomain=network_engine_domain  SubClassName=ps_output  LeftPortType=input  RightPortType=output  PseudoPeriodic=off  Frequencies=[]  VectorFormat=inherit  Unit=inherit  AffineConversion=off
  Rack orientation : sm_lib/Frames and Transforms/Rigid Transform  RotationMethod=StandardAxis  FollAlignAxisA=+X  BaseAlignAxisA=+Y  FollAlignAxisB=+Y  BaseAlignAxisB=+Z  RotationStandardAxis=+X  RotationAngle=180.0  RotationAngleUnits=deg  RotationArbitraryAxis=[0 0 1]  RotationSequenceAxes=FollowerAxes  RotationSequence=XYX  RotationSequenceAngles=[0 0 0]  RotationSequenceAnglesUnits=deg  RotationMatrix=[1 0 0; 0 1 0; 0 0 1]  Quaternion=[1 0 0 0]  TranslationMethod=None  TranslationCartesianOffset=[0 0 0]  TranslationCartesianOffsetUnits=m  TranslationStandardAxis=+Z  TranslationStandardOffset=0  TranslationStandardOffsetUnits=m  TranslationROffset=0  TranslationROffsetUnits=m  TranslationThetaOffset=0  TranslationThetaOffsetUnits=deg  TranslationZOffset=0  TranslationZOffsetUnits=m
  Rack position conversion : nesl_utility/PS-Simulink Converter  PhysicalDomain=network_engine_domain  SubClassName=ps_output  LeftPortType=input  RightPortType=output  PseudoPeriodic=off  Frequencies=[]  VectorFormat=inherit  Unit=inherit  AffineConversion=off
  Rack rotation : sm_lib/Frames and Transforms/Rigid Transform  RotationMethod=StandardAxis  FollAlignAxisA=+X  BaseAlignAxisA=+Y  FollAlignAxisB=+Y  BaseAlignAxisB=+Z  RotationStandardAxis=-Y  RotationAngle=90.0  RotationAngleUnits=deg  RotationArbitraryAxis=[0 0 1]  RotationSequenceAxes=FollowerAxes  RotationSequence=XYX  RotationSequenceAngles=[0 0 0]  RotationSequenceAnglesUnits=deg  RotationMatrix=[1 0 0; 0 1 0; 0 0 1]  Quaternion=[1 0 0 0]  TranslationMethod=None  TranslationCartesianOffset=[0 0 0]  TranslationCartesianOffsetUnits=m  TranslationStandardAxis=+Z  TranslationStandardOffset=0  TranslationStandardOffsetUnits=m  TranslationROffset=0  TranslationROffsetUnits=m  TranslationThetaOffset=0  TranslationThetaOffsetUnits=deg  TranslationZOffset=0  TranslationZOffsetUnits=m
  Rack velocity conversion : nesl_utility/PS-Simulink Converter  PhysicalDomain=network_engine_domain  SubClassName=ps_output  LeftPortType=input  RightPortType=output  PseudoPeriodic=off  Frequencies=[]  VectorFormat=inherit  Unit=inherit  AffineConversion=off
  Rigid Transform : sm_lib/Frames and Transforms/Rigid Transform  RotationMethod=RotationSequence  FollAlignAxisA=+X  BaseAlignAxisA=+Y  FollAlignAxisB=+Y  BaseAlignAxisB=+Z  RotationStandardAxis=+Z  RotationAngle=0.0  RotationAngleUnits=deg  RotationArbitraryAxis=[0 0 1]  RotationSequenceAxes=FollowerAxes  RotationSequence=ZYZ  RotationSequenceAngles=[-90 -90 0]  RotationSequenceAnglesUnits=deg  RotationMatrix=[1 0 0; 0 1 0; 0 0 1]  Quaternion=[1 0 0 0]  TranslationMethod=None  TranslationCartesianOffset=[0 0 0]  TranslationCartesianOffsetUnits=m  TranslationStandardAxis=+Z  TranslationStandardOffset=0  TranslationStandardOffsetUnits=m  TranslationROffset=0  TranslationROffsetUnits=m  TranslationThetaOffset=0  TranslationThetaOffsetUnits=deg  TranslationZOffset=0  TranslationZOffsetUnits=m
  Simulink-PS Converter : nesl_utility/Simulink-PS Converter  PhysicalDomain=network_engine_domain  SubClassName=ps_input  LeftPortType=input  RightPortType=output  PseudoPeriodic=off  Frequencies=[]  NoiseDistribution=none  NoiseParameters=[]  Unit=N  AffineConversion=off  FilteringAndDerivatives=filter  SimscapeFilterOrder=2  InputFilterTimeConstant=filter_time_constant  UdotUserProvided=0
  Single element frequency : MATLAB Function  Commented=on  TreatAsAtomicUnit=on
  Translational Multibody Interface : fl_lib/Mechanical/Multibody Interfaces/Translational Multibody Interface
  World frame : PMIOPort  Side=Left
  Contact output : PMIOPort  Port=2  Side=Right
  Rack velocity SI : Outport
  Rack position SI : Outport  Port=2
  Rack acceleration SI : Outport  Port=3
  wires:
  Rack position conversion/1 -> Single element frequency/1(cur_rack_position), Rack position SI/1  "Rack position m"
  External load input N or Nm/1 -> Simulink-PS Converter/1
  Rack velocity conversion/1 -> Rack velocity SI/1  "Rack velocity m/s"
  Rack acceleration conversion/1 -> Rack acceleration SI/1  "Rack acceleration m/ss"
  Clock/1 -> Single element frequency/2(time)
  connections:
  Mechanical Translational Reference/LConn1 -- Translational Multibody Interface/LConn2 -- Coulumb Friction/RConn1
  Rack orientation/LConn1 -- Rack anti-rotation/RConn1
  Rack Prismatic Joint1/RConn3 -- Rack velocity conversion/LConn1 -- Translational Multibody Interface/RConn1
  Rack/LConn1 -- Rigid Transform/LConn1 -- Rack orientation/RConn1 -- External Force Useful Load/RConn1
  Rack Prismatic Joint1/LConn1 -- Rack rotation/RConn1
  Grid Surface1/LConn1 -- Rigid Transform/RConn1
  Translational Multibody Interface/LConn1 -- "Rack friction converter, N"/LConn1 -- Rack Prismatic Joint1/LConn2
  Translational Multibody Interface/RConn2 -- Coulumb Friction/LConn1
  Rack rotation/LConn1 -- World frame/RConn1
  Rack Prismatic Joint1/RConn4 -- Rack acceleration conversion/LConn1
  Rack anti-rotation/LConn1 -- Rack Prismatic Joint1/RConn1
  Rack Prismatic Joint1/RConn2 -- Rack position conversion/LConn1
  Simulink-PS Converter/RConn1 -- External Force Useful Load/LConn1
  Rack Extension 0 mass/RConn1 -- Rack/LConn2
  Grid Surface1/RConn1 -- Contact output/RConn1

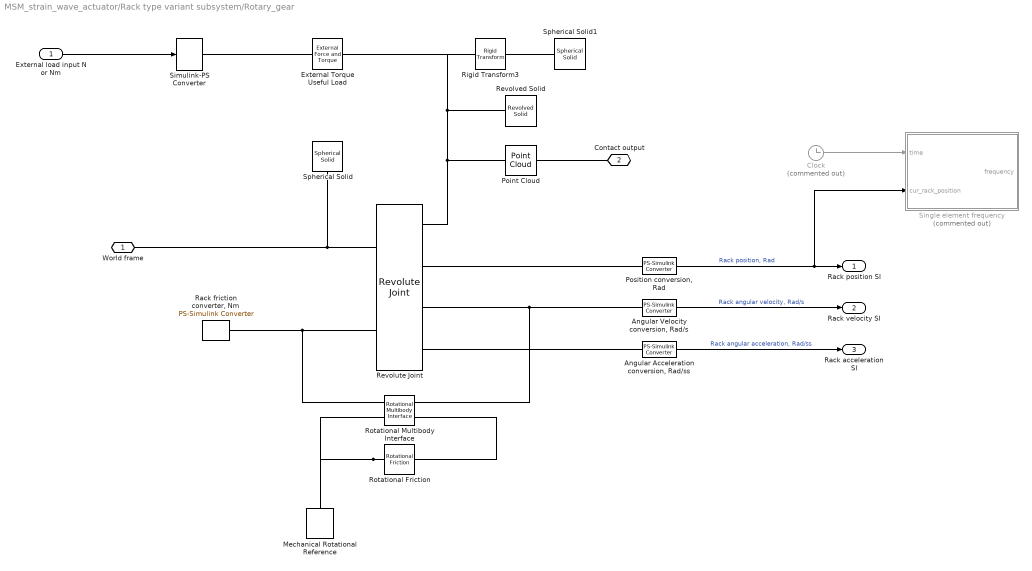
== system MSM_strain_wave_actuator/Rack type variant subsystem/Rotary_gear ==
  External load input N or Nm : Inport
  "Angular Acceleration conversion, Rad/ss" : nesl_utility/PS-Simulink Converter  PhysicalDomain=network_engine_domain  SubClassName=ps_output  LeftPortType=input  RightPortType=output  PseudoPeriodic=off  Frequencies=[]  VectorFormat=inherit  Unit=inherit  AffineConversion=off
  "Angular Velocity conversion, Rad/s" : nesl_utility/PS-Simulink Converter  PhysicalDomain=network_engine_domain  SubClassName=ps_output  LeftPortType=input  RightPortType=output  PseudoPeriodic=off  Frequencies=[]  VectorFormat=inherit  Unit=inherit  AffineConversion=off
  Clock : Clock  Commented=on
  External Torque Useful Load : sm_lib/Forces and Torques/External Force and Torque  ForceResolutionFrame=World  EnableForceX=off  EnableForceY=off  EnableForceZ=off  EnableForce=off  TorqueResolutionFrame=World  EnableTorqueX=off  EnableTorqueY=off  EnableTorqueZ=on  EnableTorque=off
  Mechanical Rotational Reference : fl_lib/Mechanical/Rotational Elements/Mechanical Rotational Reference
  Point Cloud : sm_lib/Curves and Surfaces/Point Cloud  CoordinatesMatrix=point_cloud_tooth_mat  CoordinatesMatrixUnits=m  GraphicType=MarkerCloud  GraphicSphereRadius=rotary_gear_contact_sphere_radius  GraphicSphereRadiusUnits=m  GraphicVisPropType=SimpleVisualProperties  GraphicDiffuseColor=[1 0 0]  GraphicOpacity=0.8  GraphicSpecularColor=[0.5 0.5 0.5 1.0]  GraphicAmbientColor=[0.15 0.15 0.15 1.0]  GraphicEmissiveColor=[0.0 0.0 0.0 1.0]  GraphicShininess=75
  "Position conversion, Rad" : nesl_utility/PS-Simulink Converter  PhysicalDomain=network_engine_domain  SubClassName=ps_output  LeftPortType=input  RightPortType=output  PseudoPeriodic=off  Frequencies=[]  VectorFormat=inherit  Unit=inherit  AffineConversion=off
  "Rack friction converter, Nm" : nesl_utility/PS-Simulink Converter  PhysicalDomain=network_engine_domain  SubClassName=ps_output  LeftPortType=input  RightPortType=output  PseudoPeriodic=off  Frequencies=[]  VectorFormat=inherit  Unit=inherit  AffineConversion=off
  Revolute Joint : sm_lib/Joints/Revolute Joint  JointMode=Normal  SenseConstraintForce=off  SenseConstraintForceX=off  SenseConstraintForceY=off  SenseConstraintForceZ=off  SenseConstraintTorque=off  SenseConstraintTorqueX=off  SenseConstraintTorqueY=off  SenseConstraintTorqueZ=off  SenseTotalForce=off  SenseTotalForceX=off  SenseTotalForceY=off  SenseTotalForceZ=off  SenseTotalTorque=off  SenseTotalTorqueX=off  SenseTotalTorqueY=off  SenseTotalTorqueZ=off  CompositeWrenchDir=FollowerOnBase  CompositeWrenchFrame=BaseFrame  EquilibriumPosition=0  EquilibriumPositionUnits=deg  SpringStiffness=0  SpringStiffnessUnits=N*m/deg  DampingCoefficient=0  DampingCoefficientUnits=N*m/(deg/s)  TorqueActuationMode=InputTorque  MotionActuationMode=ComputedMotion  SensePosition=on  SenseVelocity=on  SenseAcceleration=on  SenseTorqueForce=off  SenseLowerLimitTorqueForce=off  SenseUpperLimitTorqueForce=off  LowerLimitSpecify=off  LowerLimitBound=-90  LowerLimitBoundUnits=deg  LowerLimitStiffness=1e4  LowerLimitStiffnessUnits=N*m/deg  LowerLimitDamping=10  LowerLimitDampingUnits=N*m/(deg/s)  LowerLimitTransitionRegionWidth=0.1  LowerLimitTransitionRegionWidthUnits=deg  UpperLimitSpecify=off  UpperLimitBound=90  UpperLimitBoundUnits=deg  UpperLimitStiffness=1e4  UpperLimitStiffnessUnits=N*m/deg  UpperLimitDamping=10  UpperLimitDampingUnits=N*m/(deg/s)  UpperLimitTransitionRegionWidth=0.1  UpperLimitTransitionRegionWidthUnits=deg  PositionTargetSpecify=on  PositionTargetPriority=High  PositionTargetValue=rack_initial_position  PositionTargetValueUnits=rad  VelocityTargetSpecify=on  VelocityTargetPriority=High  VelocityTargetValue=rack_initial_velocity  VelocityTargetValueUnits=rad/s
  Revolved Solid : sm_lib/Body Elements/Revolved Solid  GraphicAmbientColor=[0.15 0.15 0.15 1.0]  BasedOnType=Mass  CenterOfMass=[0 0 0]  CenterOfMassUnits=m  GraphicDiffuseColor=[1.0 0.8 0.0]  ExportConvexHullGeometry=off  Density=1000  DensityUnits=kg/m^3  DoExposeReferenceFrame=on  GraphicEmissiveColor=[0.0 0.0 0.0 1.0]  ExportEntireGeometry=off  SerializedFrames=<Frames/>  MarkerShape=Sphere  MarkerSize=10  GraphicType=FromGeometry  InertiaType=CalculateFromGeometry  Mass=tooth_disk_mass+useful_mass  MassUnits=kg  MomentsOfInertia=[1 1 1]  MomentsOfInertiaUnits=kg*m^2  GraphicOpacity=0.8  ProductsOfInertia=[0 0 0]  ProductsOfInertiaUnits=kg*m^2  RevolutionCrossSection=disk_cross_section  RevolutionCrossSectionUnits=m  RevolutionAngle=180  RevolutionAngleUnits=deg  RevolutionExtent=Full  GraphicShininess=75  GraphicSpecularColor=[0.5 0.5 0.5 1.0]  GraphicVisPropType=SimpleVisualProperties
  Rigid Transform3 : sm_lib/Frames and Transforms/Rigid Transform  TranslationMethod=Cartesian  TranslationStandardOffset=0  TranslationStandardOffsetUnits=m  TranslationStandardAxis=+X  TranslationCartesianOffset=[disk_diameter/2 0 -disk_height]  TranslationCartesianOffsetUnits=m  TranslationROffset=0  TranslationROffsetUnits=m  TranslationZOffset=0  TranslationZOffsetUnits=m  TranslationThetaOffset=0  TranslationThetaOffsetUnits=deg  RotationMethod=None  RotationAngleUnits=deg  RotationStandardAxis=+Z  RotationAngle=0.0  RotationArbitraryAxis=[0 0 1]  FollAlignAxisA=+X  BaseAlignAxisA=+Y  FollAlignAxisB=+Y  BaseAlignAxisB=+Z  RotationSequenceAxes=FollowerAxes  RotationSequence=XYX  RotationSequenceAngles=[0 0 0]  RotationSequenceAnglesUnits=deg  RotationMatrix=[1 0 0; 0 1 0; 0 0 1]  Quaternion=[1 0 0 0]
  Rotational Friction : fl_lib/Mechanical/Rotational Elements/Rotational Friction  brkwy_trq=rotational_rack_coulumb_friction * (1 + 1e-5) N*m  brkwy_vel=1e-2 rad/s  Col_trq=rotational_rack_coulumb_friction N*m  visc_coef=rotational_contact_coeff_kinetic_friction N*m*s/rad  w_specify=off  w_priority=None  w=0 rad/s  w_nominal_specify=off  w_nominal_unit=rad/s  w_nominal_value=1  t_specify=off  t_priority=None  t=0 N*m  t_nominal_specify=off  t_nominal_unit=N*m  t_nominal_value=1
  Rotational Multibody Interface : fl_lib/Mechanical/Multibody Interfaces/Rotational Multibody Interface
  Simulink-PS Converter : nesl_utility/Simulink-PS Converter  PhysicalDomain=network_engine_domain  SubClassName=ps_input  LeftPortType=input  RightPortType=output  PseudoPeriodic=off  Frequencies=[]  NoiseDistribution=none  NoiseParameters=[]  Unit=N*m  AffineConversion=off  FilteringAndDerivatives=filter  SimscapeFilterOrder=2  InputFilterTimeConstant=filter_time_constant  UdotUserProvided=0
  Single element frequency : MATLAB Function  Commented=on  TreatAsAtomicUnit=on
  Spherical Solid : sm_lib/Body Elements/Spherical Solid  GraphicAmbientColor=[0.15 0.15 0.15 1.0]  BasedOnType=Density  CenterOfMass=[0 0 0]  CenterOfMassUnits=m  GraphicDiffuseColor=[1.0 0.2 0.2]  Density=1000  DensityUnits=kg/m^3  DoExposeReferenceFrame=on  GraphicEmissiveColor=[0.0 0.0 0.0 1.0]  ExportEntireGeometry=off  SerializedExposedGeometries=<ExposedGeometries/>  SerializedFrames=<Frames/>  MarkerShape=Sphere  MarkerSize=10  GraphicType=FromGeometry  InertiaType=CalculateFromGeometry  Mass=1  MassUnits=kg  MomentsOfInertia=[1 1 1]  MomentsOfInertiaUnits=kg*m^2  GraphicOpacity=1.0  ProductsOfInertia=[0 0 0]  ProductsOfInertiaUnits=kg*m^2  GraphicShininess=75  GraphicSpecularColor=[0.5 0.5 0.5 1.0]  SphereRadius=4e-4  SphereRadiusUnits=m  GraphicVisPropType=SimpleVisualProperties
  Spherical Solid1 : sm_lib/Body Elements/Spherical Solid  GraphicAmbientColor=[0.15 0.15 0.15 1.0]  BasedOnType=Mass  CenterOfMass=[0 0 0]  CenterOfMassUnits=m  GraphicDiffuseColor=[0.2 0.8 0.0]  Density=1000  DensityUnits=kg/m^3  DoExposeReferenceFrame=on  GraphicEmissiveColor=[0.0 0.0 0.0 1.0]  ExportEntireGeometry=off  SerializedExposedGeometries=<ExposedGeometries/>  SerializedFrames=<Frames/>  MarkerShape=Sphere  MarkerSize=10  GraphicType=FromGeometry  InertiaType=CalculateFromGeometry  Mass=1e-10  MassUnits=kg  MomentsOfInertia=[1 1 1]  MomentsOfInertiaUnits=kg*m^2  GraphicOpacity=1.0  ProductsOfInertia=[0 0 0]  ProductsOfInertiaUnits=kg*m^2  GraphicShininess=75  GraphicSpecularColor=[0.5 0.5 0.5 1.0]  SphereRadius=3e-4  SphereRadiusUnits=m  GraphicVisPropType=SimpleVisualProperties
  World frame : PMIOPort  Side=Left
  Contact output : PMIOPort  Port=2  Side=Right
  Rack position SI : Outport
  Rack velocity SI : Outport  Port=2
  Rack acceleration SI : Outport  Port=3
  wires:
  "Angular Velocity conversion, Rad/s"/1 -> Rack velocity SI/1  "Rack angular velocity, Rad/s"
  "Angular Acceleration conversion, Rad/ss"/1 -> Rack acceleration SI/1  "Rack angular acceleration, Rad/ss"
  External load input N or Nm/1 -> Simulink-PS Converter/1
  "Position conversion, Rad"/1 -> Rack position SI/1, Single element frequency/2(cur_rack_position)  "Rack position, Rad"
  Clock/1 -> Single element frequency/1(time)
  connections:
  Point Cloud/LConn1 -- Revolute Joint/RConn1 -- Revolved Solid/RConn1 -- External Torque Useful Load/RConn1 -- Rigid Transform3/LConn1
  "Position conversion, Rad"/LConn1 -- Revolute Joint/RConn2
  Point Cloud/RConn1 -- Contact output/RConn1
  Spherical Solid/RConn1 -- World frame/RConn1 -- Revolute Joint/LConn1
  Spherical Solid1/RConn1 -- Rigid Transform3/RConn1
  "Rack friction converter, Nm"/LConn1 -- Rotational Multibody Interface/LConn1 -- Revolute Joint/LConn2
  Rotational Multibody Interface/RConn1 -- Revolute Joint/RConn3 -- "Angular Velocity conversion, Rad/s"/LConn1
  "Angular Acceleration conversion, Rad/ss"/LConn1 -- Revolute Joint/RConn4
  Rotational Friction/LConn1 -- Mechanical Rotational Reference/LConn1 -- Rotational Multibody Interface/LConn2
  Rotational Friction/RConn1 -- Rotational Multibody Interface/RConn2
  External Torque Useful Load/LConn1 -- Simulink-PS Converter/RConn1

== system MSM_strain_wave_actuator/controller/Check if actuator halted or overloaded or reached max position ==
  is_load_applied : Inport
  cur_rack_position : Inport  Port=2
  Abs : Abs  Commented=on  SaturateOnIntegerOverflow=off
  Check sim stop conditions : MATLAB Function  TreatAsAtomicUnit=on
  Clock1 : Clock
  Compare To Constant : simulink/Logic and Bit Operations/Compare To Constant  relop=>=  const=0.5  OutDataTypeStr=boolean
  Compare To Constant1 : simulink/Logic and Bit Operations/Compare To Constant  relop=>=  const=0.5  OutDataTypeStr=boolean
  Constant : Constant  Commented=on  Value=rack_initial_position
  DISABLED FOR NN TRAINING Stop Simulation : Stop  Commented=on
  Delay : Delay  DelayLength=1  InitialCondition=NaN
  Delay1 : Delay
  Mean : spsMeanLib/Mean  Commented=on  Freq=1 / (SIMULATION_TIME * 0.05)  Vinit=0  Ts=0
  Save scalar result : Subsystem  TreatAsAtomicUnit=on
  stop_sim_code : Outport
  wires:
  Compare To Constant1/1 -> Check sim stop conditions/1(is_load_applied)
  Clock1/1 -> Check sim stop conditions/2(time)
  is_load_applied/1 -> Compare To Constant1/1
  Abs/1 -> Mean/1
  Check sim stop conditions/1(stop_sim_code) -> Delay1/1, stop_sim_code/1
  cur_rack_position/1 -> Check sim stop conditions/3(rack_cur_pos)
  Delay/1 -> Check sim stop conditions/4(memory_pos)
  Check sim stop conditions/3(out_pos) -> Delay/1
  Compare To Constant/1 -> DISABLED FOR NN TRAINING Stop Simulation/1, Save scalar result/Enable
  Delay1/1 -> Save scalar result/1(stop_sim_code), Compare To Constant/1

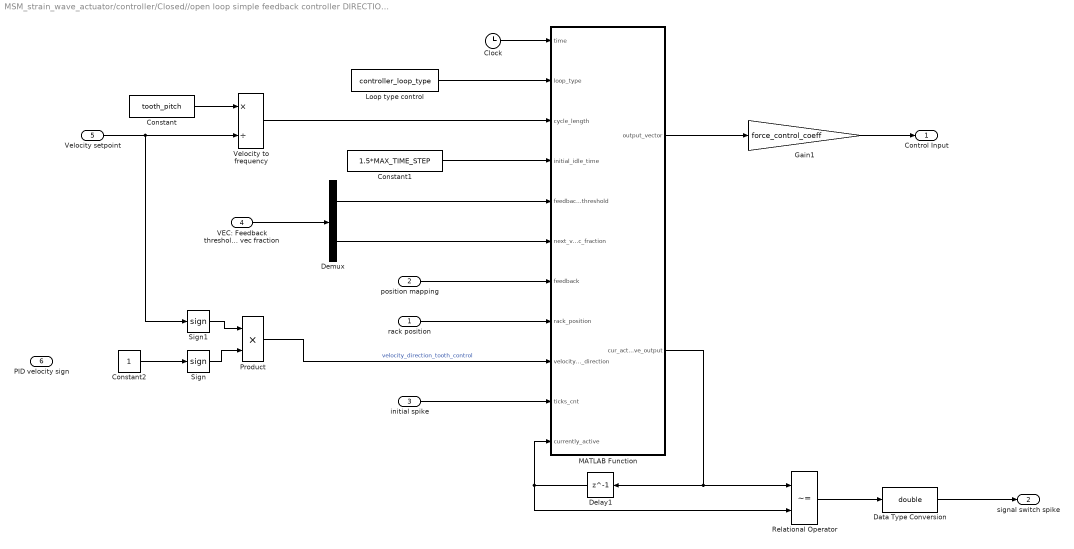
== system MSM_strain_wave_actuator/controller/Closed//open loop simple feedback controller DIRECTION SWITCH IS BLOCKED!!!! ==
  rack position : Inport
  position mapping : Inport  Port=2
  initial spike : Inport  Port=3
  VEC: Feedback threshold and next vec fraction : Inport  Port=4
  Velocity setpoint : Inport  Port=5
  PID velocity sign : Inport  Port=6
  Clock : Clock
  Constant : Constant  Value=tooth_pitch
  Constant1 : Constant  Value=1.5*MAX_TIME_STEP
  Constant2 : Constant
  Data Type Conversion : DataTypeConversion  OutDataTypeStr=double  RndMeth=Round  SaturateOnIntegerOverflow=off
  Delay1 : Delay  DelayLength=1  InitialCondition=1
  Demux : Demux  Outputs=2
  Gain1 : Gain  Gain=force_control_coeff
  Loop type control : Constant  Value=controller_loop_type
  MATLAB Function : MATLAB Function  TreatAsAtomicUnit=on
  Product : Product
  Relational Operator : RelationalOperator  Operator=~=  OutDataTypeStr=boolean  RndMeth=Simplest  InputSameDT=off
  Sign : Signum
  Sign1 : Signum
  Velocity to frequency : Product  Inputs=*/
  Control Input : Outport
  signal switch spike : Outport  Port=2
  wires:
  Constant1/1 -> MATLAB Function/4(initial_idle_time)
  Velocity to frequency/1 -> MATLAB Function/3(cycle_length)
  Loop type control/1 -> MATLAB Function/2(loop_type)
  MATLAB Function/1(output_vector) -> Gain1/1
  rack position/1 -> MATLAB Function/8(rack_position)
  MATLAB Function/2(cur_active_output) -> Delay1/1, Relational Operator/1
  Delay1/1 -> Relational Operator/2, MATLAB Function/11(currently_active)
  Clock/1 -> MATLAB Function/1(time)
  initial spike/1 -> MATLAB Function/10(ticks_cnt)
  position mapping/1 -> MATLAB Function/7(feedback)
  Gain1/1 -> Control Input/1
  Constant/1 -> Velocity to frequency/1
  Demux/1 -> MATLAB Function/5(feedback_threshold)
  Demux/2 -> MATLAB Function/6(next_vec_fraction)
  VEC: Feedback threshold and next vec fraction/1 -> Demux/1
  Relational Operator/1 -> Data Type Conversion/1
  Data Type Conversion/1 -> signal switch spike/1
  Sign/1 -> Product/2
  Sign1/1 -> Product/1
  Product/1 -> MATLAB Function/9(velocity_direction)  "velocity_direction_tooth_control"
  Constant2/1 -> Sign/1
  Velocity setpoint/1 -> Sign1/1, Velocity to frequency/2
